simulink model "es1sim"  (R2023b)
settings: Solver=VariableStepAuto  StartTime=0.0  StopTime=Tfin  RelTol=1e-3
values from neighbouring files (symbols this model uses):
  IJ = inv(J)    [es1.m]    (also in es2.m; es3.m)
  J = [937.5 833.3 270.8]    [dyn_kin_quat.m]    (also in es1.m = diag([937.5, 833.3, 270.8]); es2.m = diag([937.5, 833.3, 270.8]); es3.m = diag([937.5, 833.3, 270.8]); euler_eq.m = [400 50 150])
  M = [0,0,0]'    [es1.m]    (also in es2.m = [0 0 0]; es3.m = [0 0 0])
  q0 = [1,0,0,0]'    [es1.m]
  w0 = [1,0.1,0]'    [es1.m]    (also in es2.m; es3.m)
libraries: vrlib x1
settings Model: Creator=luigi  LastModifiedBy=luigi

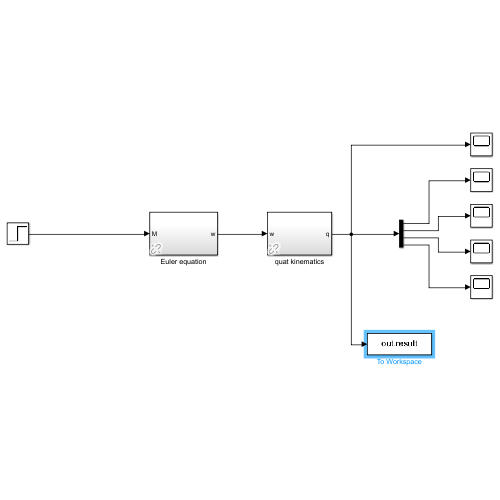
[thumbnail: Simulink's stored preview of the top-level diagram]
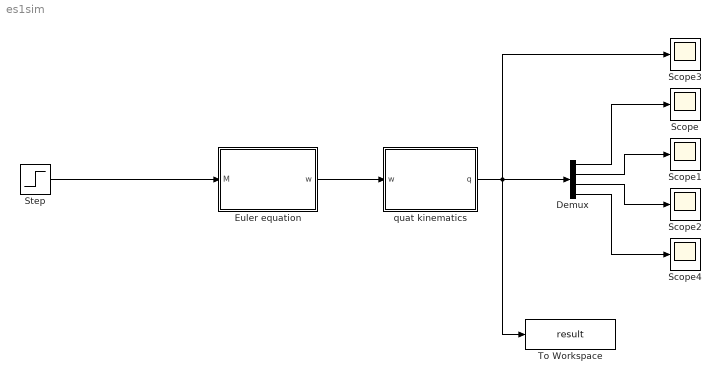
== system es1sim ==
  Demux : Demux
  Euler equation : Subsystem  AncestorBlock=lib_rotations_2014/Euler equation
  Scope{,1..4} (5 alike) : Scope
  Step : Step  After=M  SampleTime=0
  To Workspace : ToWorkspace  VariableName=result  SaveFormat=Timeseries  SampleTime=-1
  quat kinematics : Subsystem  AncestorBlock=lib_rotations_2014/quat kinematics
  wires:
  Euler equation/1(w) -> quat kinematics/1(w)
  quat kinematics/1(q) -> To Workspace/1, Scope3/1, Demux/1
  Demux/1 -> Scope/1
  Demux/2 -> Scope1/1
  Demux/3 -> Scope2/1
  Demux/4 -> Scope4/1
  Step/1 -> Euler equation/1(M)

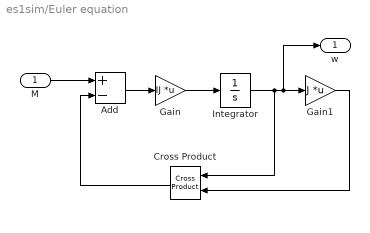
== system es1sim/Euler equation ==
  M : Inport
  Add : Sum  Inputs=+-
  Cross Product : vrlib/Utilities/Cross Product
  Gain : Gain  Gain=IJ  Multiplication=Matrix(K*u)
  Gain1 : Gain  Gain=J  Multiplication=Matrix(K*u)
  Integrator : Integrator  InitialCondition=w0
  w : Outport  VectorParamsAs1DForOutWhenUnconnected=off
  wires:
  Cross Product/1 -> Add/2
  Add/1 -> Gain/1
  Gain1/1 -> Cross Product/2
  Gain/1 -> Integrator/1
  Integrator/1 -> Gain1/1, w/1, Cross Product/1
  M/1 -> Add/1

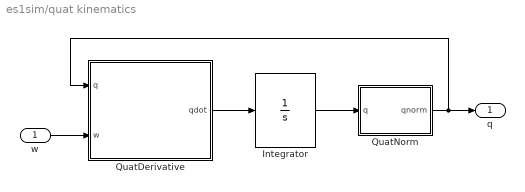
== system es1sim/quat kinematics ==
  w : Inport  PortDimensions=3
  Integrator : Integrator  InitialCondition=q0
  QuatDerivative : MATLAB Function  TreatAsAtomicUnit=on
  QuatNorm : MATLAB Function  TreatAsAtomicUnit=on
  q : Outport  PortDimensions=4  VectorParamsAs1DForOutWhenUnconnected=off
  wires:
  w/1 -> QuatDerivative/2(w)
  QuatDerivative/1(qdot) -> Integrator/1
  QuatNorm/1(qnorm) -> q/1, QuatDerivative/1(q)
  Integrator/1 -> QuatNorm/1(q)

== matlab function es1sim/quat kinematics/QuatDerivative ==
  data: q input; qdot output; w input
function qdot= QuatDerivative(q,w)
%#codegen
omegaq=[0; w];
Q=[q(1) -q(2) -q(3) -q(4);
    q(2) q(1) -q(4) q(3);
    q(3) q(4) q(1) -q(2);
    q(4) -q(3) q(2) q(1)];
qdot=Q*omegaq/2;

== matlab function es1sim/quat kinematics/QuatNorm ==
  data: q input; qnorm output
function qnorm = QuatNorm(q)
%#codegen
qnorm=zeros(4,1);
q2=sqrt(q'*q);
qnorm=q/q2;
